simulink model "sim_grzejnikowa_model_bojlera_domu"  (R2021b)
settings: Solver=VariableStepAuto  StartTime=0.0  StopTime=10.0  MaxStep=5  RelTol=1e-3
undefined symbols (not defined in the file): dRz_g, k, skok_czas2, T0_klasyczna, T_klasyczna
settings Model: Creator=adams  LastModifiedBy=adams

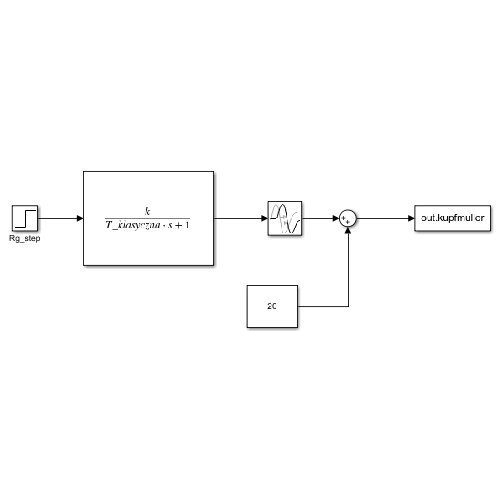
[thumbnail: Simulink's stored preview of the top-level diagram]
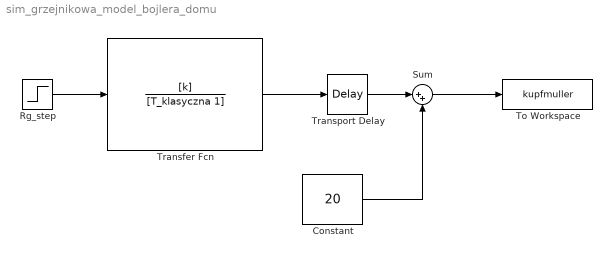
== system sim_grzejnikowa_model_bojlera_domu ==
  Constant : Constant  Value=20
  Rg_step : Step  Time=skok_czas2  After=dRz_g  SampleTime=0
  Sum : Sum  Inputs=|++
  To Workspace : ToWorkspace  VariableName=kupfmuller  SampleTime=-1
  Transfer Fcn : TransferFcn  Numerator=[k]  Denominator=[T_klasyczna 1]
  Transport Delay : TransportDelay  DelayTime=T0_klasyczna  BufferSize=32768
  wires:
  Constant/1 -> Sum/2
  Transport Delay/1 -> Sum/1
  Rg_step/1 -> Transfer Fcn/1
  Transfer Fcn/1 -> Transport Delay/1
  Sum/1 -> To Workspace/1
